simulink model "Lab_05_ShortCircuitTestofaTransformers"  (R2024b)
settings: Solver=VariableStepAuto  StartTime=0.0  StopTime=1  RelTol=1e-3
libraries: spsRMSLib x2, spsACVoltageSourceLib x1, spsCurrentMeasurementLib x1, spsLinearTransformerLib x1, eePowerMeasurement x1, spsVoltageMeasurementLib x1, sps_lib x1
settings Model: Creator=yashr  LastModifiedBy=yashr

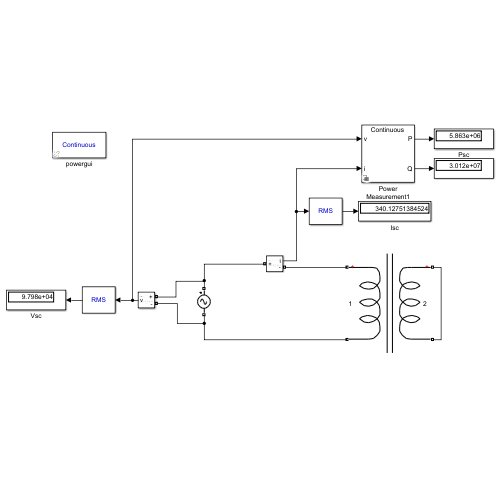
[thumbnail: Simulink's stored preview of the top-level diagram]
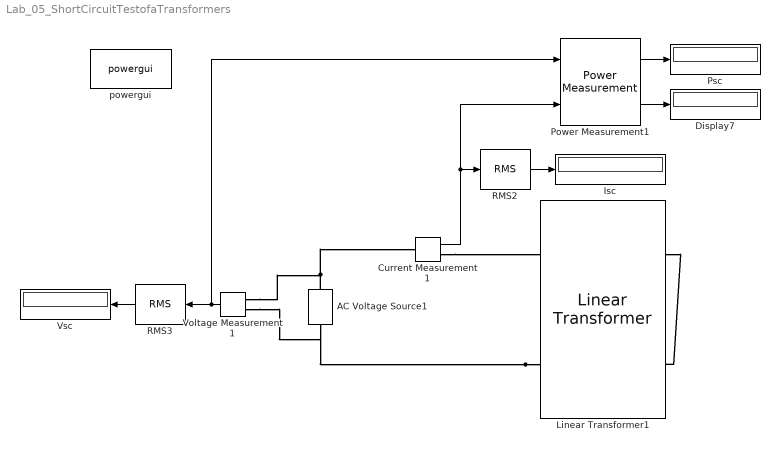
== system Lab_05_ShortCircuitTestofaTransformers ==
  AC Voltage Source1 : spsACVoltageSourceLib/AC Voltage Source  Amplitude=(7.35e+05)*sqrt(2)*0.133305  Phase=0  Frequency=50  SampleTime=0  Measurements=None  BusType=swing  Pref=10e3  Qref=0  Qmin=-inf  Qmax=+inf
  Current Measurement1 : spsCurrentMeasurementLib/Current Measurement  PhasorSimulation=off  OutputType=Complex  PSBequivalent=0
  Display7 : Display
  Isc : Display
      settings: Format=decimal (Stored Integer)  Decimation=3
  Linear Transformer1 : spsLinearTransformerLib/Linear Transformer  UNITS=SI  NominalPower=[ 250e6 50 ]  winding1=[7.35e+05 4.3218 0.45856]  winding2=[3.15e+05 0.7938 0.084225]  ThreeWindings=off  winding3=[3.15e+05 0.7938 0.084225]  RmLm=[1.0804e+06 2866]  Measurements=None  DataType=on
  Power Measurement1 : eePowerMeasurement/Power Measurement  LabelModeActiveChoice=Continuous  F=60  K=[1]  Ts=0
  Psc : Display
  RMS2 : spsRMSLib/RMS  TrueRMS=on  Freq=50  RMSInit=120  Ts=0
  RMS3 : spsRMSLib/RMS  TrueRMS=on  Freq=50  RMSInit=120  Ts=0
  Voltage Measurement1 : spsVoltageMeasurementLib/Voltage Measurement  PhasorSimulation=off  OutputType=Complex  PSBequivalent=0
  Vsc : Display
  powergui : sps_lib/powergui  Priority=1  SimulationMode=Continuous  SampleTime=50e-6  frequency=60  Iterations=50  frequencyindice=50  Pbase=100e6  ErrMax=1e-4  UnitsV=kV  UnitsW=MW  buscounter=0  FunctionMessages=off  echomessages=off  EnableUseOfTLC=off  CurrentSourceSwitches=off  DisableSnubberDevices=off  DisableRonSwitches=off  DisableVfSwitches=off  DisplayEquations=off  AutomaticDiscreteSolvers=off  SolverType=Tustin/Backward Euler (TBE)  Interpol=off  ExternalGateDelay=off  methode=off  Ts=100  x0status=blocks  SPID=on  SwTol=0  HookPort=off  NonlinearTolerance=1e-4  nMaxIteration=100  ContinueOnMaxIteration=off  RestoreLinks=warning  ResistiveCurrentMeasurement=off  Frange=[0:2:500]  Ylog=off  Xlog=on  ShowGrid=off  save=off  variable=ZData  structure=0  ZoomFFT=off  StartTime=0.0  cycles=1  DisplayStyle=1  fundamental=60  FreqAxis=off  MaxFrequency=1000  frequencyindicesteady=1  RmsSteady=1  display=off
  wires:
  RMS3/1 -> Vsc/1
  Power Measurement1/1 -> Psc/1
  RMS2/1 -> Isc/1
  Voltage Measurement1/1 -> RMS3/1, Power Measurement1/1
  Current Measurement1/1 -> RMS2/1, Power Measurement1/2
  Power Measurement1/2 -> Display7/1
  connections:
  Voltage Measurement1/LConn1 -- AC Voltage Source1/RConn1 -- Current Measurement1/LConn1
  Linear Transformer1/LConn2 -- AC Voltage Source1/LConn1 -- Voltage Measurement1/LConn2
  Current Measurement1/RConn1 -- Linear Transformer1/LConn1
  Linear Transformer1/RConn1 -- Linear Transformer1/RConn2
